simulink library "cdsOscSetPhase"  (Simulink 8.0)
settings: Solver=ode45  SolverMode=SingleTasking  StartTime=0.0  StopTime=10.0  RelTol=1e-3
settings Model: Creator=maronsso  LastModifiedBy=controls

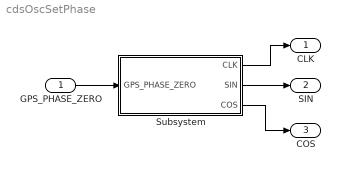
== system cdsOscSetPhase ==
  GPS_PHASE_ZERO : Inport
  Subsystem : Subsystem  Description=ADL=OSC.adl
  CLK : Outport
  SIN : Outport  Port=2
  COS : Outport  Port=3
  wires:
  Subsystem/1(CLK) -> CLK/1
  Subsystem/2(SIN) -> SIN/1
  Subsystem/3(COS) -> COS/1
  GPS_PHASE_ZERO/1 -> Subsystem/1("GPS_PHASE_ZERO ")

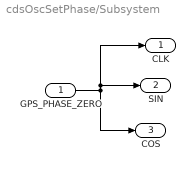
== system cdsOscSetPhase/Subsystem ==
  "GPS_PHASE_ZERO " : Inport
  CLK : Outport
  SIN : Outport  Port=2
  COS : Outport  Port=3
  wires:
  "GPS_PHASE_ZERO "/1 -> CLK/1, SIN/1, COS/1
